simulink model "l1_1"  (R2014b)
settings: Solver=ode45  StartTime=0.0  StopTime=10.0  RelTol=1e-3
settings Model: Creator=Admin  LastModifiedBy=Admin

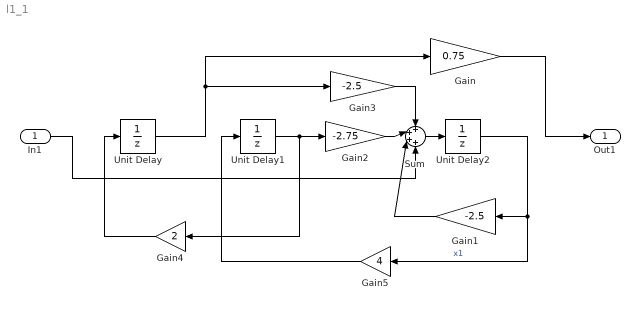
== system l1_1 ==
  In1 : Inport
  Gain : Gain  Gain=0.75
  Gain1 : Gain  Gain=-2.5
  Gain2 : Gain  Gain=-2.75
  Gain3 : Gain  Gain=-2.5
  Gain4 : Gain  Gain=2
  Gain5 : Gain  Gain=4
  Sum : Sum  Inputs=++++
  Unit Delay : UnitDelay  SampleTime=-1
  Unit Delay1 : UnitDelay  SampleTime=-1
  Unit Delay2 : UnitDelay  SampleTime=-1
  Out1 : Outport
  wires:
  Unit Delay2/1 -> Gain1/1, Gain5/1  "x1"
  Unit Delay1/1 -> Gain4/1, Gain2/1
  Sum/1 -> Unit Delay2/1
  Unit Delay/1 -> Gain/1, Gain3/1
  Gain1/1 -> Sum/3
  Gain2/1 -> Sum/2
  Gain3/1 -> Sum/1
  In1/1 -> Sum/4
  Gain5/1 -> Unit Delay1/1
  Gain4/1 -> Unit Delay/1
  Gain/1 -> Out1/1
